simulink model "un"  (Simulink 7.9)
settings: Solver=ode45  StartTime=0.0  StopTime=10.0  RelTol=1e-3
settings Model: Creator=aziemba  LastModifiedBy=aziemba

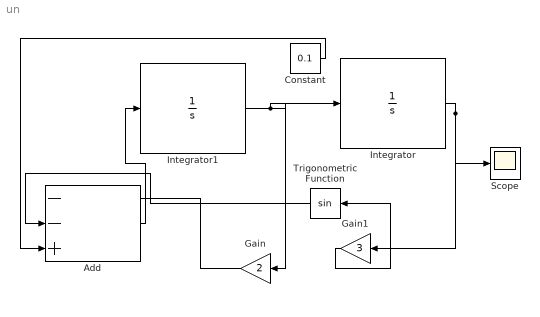
== system un ==
  Add : Sum  Inputs=--+
  Constant : Constant  Value=0.1
  Gain : Gain  Gain=2
  Gain1 : Gain  Gain=3
  Integrator : Integrator
  Integrator1 : Integrator  InitialCondition=2
  Scope : Scope
  Trigonometric Function : Trigonometry
  wires:
  Integrator1/1 -> Integrator/1, Gain/1
  Add/1 -> Integrator1/1
  Integrator/1 -> Gain1/1, Scope/1
  Gain/1 -> Add/1
  Gain1/1 -> Trigonometric Function/1
  Constant/1 -> Add/3
  Trigonometric Function/1 -> Add/2
